simulink model "es_motore_con_controllo_velocita"  (Simulink 8.3)
settings: Solver=ode45  StartTime=0.0  StopTime=20  RelTol=1e-6
values from neighbouring files (symbols this model uses):
  Td_amp = 0.05    [ES4_1.m]
undefined symbols (not defined in the file or in its folder): Kc
libraries: cstblocks x2
settings Model: Creator=Taragna  LastModifiedBy=Taragna  ExtModeTrigMode=oneshot  ExtModeArmWhenConnect=off
settings DataIOCC: LimitDataPoints=off
settings OptimizationCC: BlockReduction=off  BooleanDataType=off
settings DebuggingCC: SaveWithParameterizedLinksMsg=none  SignalResolutionControl=TryResolveAllWithWarning  SolverPrmCheckMsg=none  MultiTaskDSMMsg=warning  MultiTaskCondExecSysMsg=none  StateNameClashWarn=none
settings HardwareCC: TargetUnknown=on
settings RTWCC: IncludeERTFirstTime=on

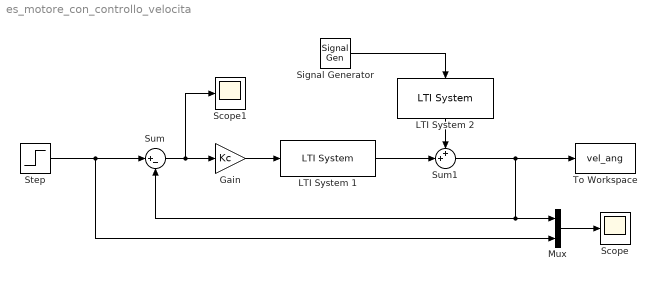
== system es_motore_con_controllo_velocita ==
  Gain : Gain  Gain=Kc  OutDataTypeStr=Inherit: Same as input  ParamDataTypeStr=Inherit: Same as input
  LTI System 1 : cstblocks/LTI System  sys=F1  IC=[0]
  LTI System 2 : cstblocks/LTI System  sys=F2  IC=[0]
  Mux : Mux  Inputs=2
  Scope : Scope
  Scope1 : Scope
  Signal Generator : SignalGenerator  WaveForm=square  Amplitude=Td_amp  Frequency=0.1
  Step : Step  Time=0  SampleTime=0
  Sum : Sum  Inputs=|+-  SaturateOnIntegerOverflow=on  InputSameDT=on  OutDataTypeStr=Inherit: Same as first input
  Sum1 : Sum  Inputs=++|  SaturateOnIntegerOverflow=on  InputSameDT=on  OutDataTypeStr=Inherit: Same as first input
  To Workspace : ToWorkspace  VariableName=vel_ang  SampleTime=-1
  wires:
  Step/1 -> Sum/1, Mux/2
  Mux/1 -> Scope/1
  Gain/1 -> LTI System 1/1
  LTI System 1/1 -> Sum1/2
  LTI System 2/1 -> Sum1/1
  Sum1/1 -> To Workspace/1, Sum/2, Mux/1
  Signal Generator/1 -> LTI System 2/1
  Sum/1 -> Gain/1, Scope1/1
